simulink model "MotorJaulaArdillav2"  (R2023a)
settings: Solver=ode23s  StartTime=0.0  StopTime=1517  MaxStep=1e-3  RelTol=1e-3
PostLoadFcn:
  | load('NewCycleFTP75.mat')
  | 
  | Vel=Cycle(:,1);
  | Acc=Cycle(:,2);
InitFcn:
  | load('NewCycleFTP75.mat')
  | 
  | Vel=Cycle(:,1);
  | Acc=Cycle(:,2);
undefined symbols (not defined in the file or in its folder): sizecont
libraries: spsControlledVoltageSourceLib x3, spsAsynchronousMachineSIUnitsLib x2, dspswit3 x1, spsGroundLib x1, spsPower3phInstantaneousLib x1, spsThreePhaseVIMeasurementLib x1, spspowerguiLib x1
settings Model: SimulationMode=accelerator  Creator=ONTIBON  LastModifiedBy=Julian
settings SolverCC: ZeroCrossAlgorithm=Adaptive
settings OptimizationCC: ReuseModelBlockBuffer=off
settings DebuggingCC: IgnoredZcDiagnostic=error

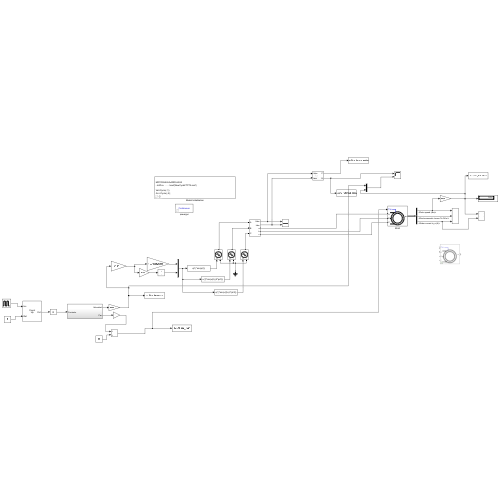
[thumbnail: Simulink's stored preview of the top-level diagram]
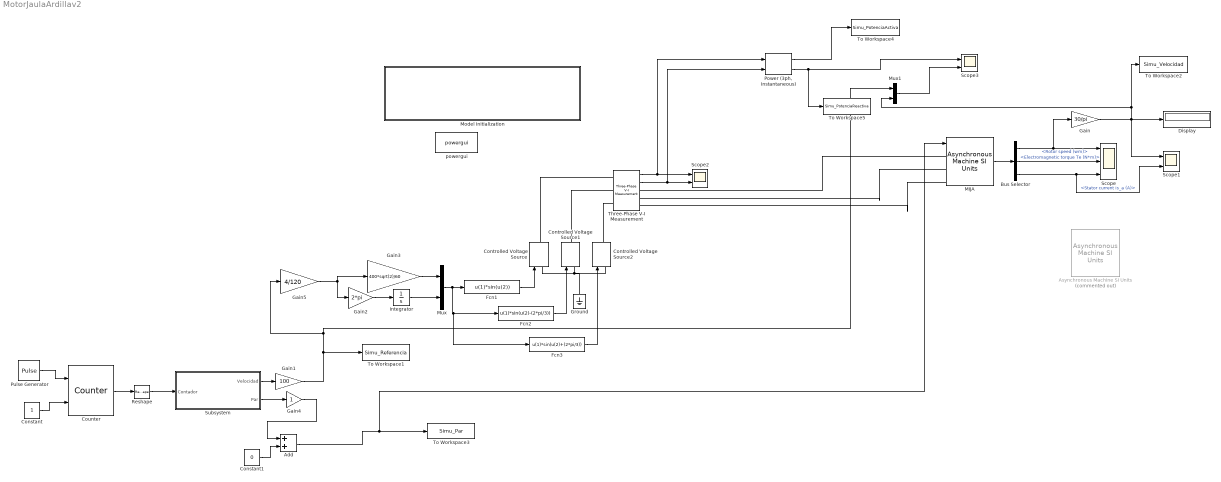
== system MotorJaulaArdillav2 ==
  Add : Sum
  Asynchronous Machine SI Units : spsAsynchronousMachineSIUnitsLib/Asynchronous Machine SI Units  Commented=on  RotorType=Squirrel-cage  PresetModel=No  MechanicalLoad=Torque Tm  ShowDetailedParameters=on  ReferenceFrame=Rotor  Units=SI  MeasurementBus=off  NominalParameters=[1.845e+04 400 50]  VoltageRatio=1  Stator=[0.5968 0.0003495]  Rotor=[0.6258 0.005473]  Cage1=[0.4155 0.002066]  Cage2=[0.4168 0.0003495]  Lm=0.0354  Mechanical=[0.05 0.005879 2]  PolePairs=2  InitialConditions=[1 0 0 0 0 0 0 0]  SimulateSaturation=off  Saturation=[14.03593122, 27.81365428, 53.79336849, 72.68890987, 97.98006896, 148.6815601, 215.7428561, 302.9841135, 428.7778367 ; 230, 322, 414, 460, 506, 552, 598, 644, 690]  LoadFlowParameters=1492000  TsPowergui=0  TsBlock=-1  IterativeModel=Trapezoidal non iterative  IterativeDiscreteModel=Trapezoidal non iterative  Pmec=1.492e+006
  Bus Selector : BusSelector  OutputSignals=Mechanical.Rotor speed (wm),Mechanical.Electromagnetic torque Te (N*m),Stator measurements.Stator current is_a (A)
  Constant : Constant
  Constant1 : Constant  Value=0
  Controlled Voltage Source : spsControlledVoltageSourceLib/Controlled Voltage Source  Initialize=on  Source_Type=AC  Amplitude=0  Phase=0  Frequency=0  Measurements=None
  Controlled Voltage Source1 : spsControlledVoltageSourceLib/Controlled Voltage Source  Initialize=on  Source_Type=AC  Amplitude=0  Phase=0  Frequency=0  Measurements=None
  Controlled Voltage Source2 : spsControlledVoltageSourceLib/Controlled Voltage Source  Initialize=on  Source_Type=AC  Amplitude=0  Phase=0  Frequency=0  Measurements=None
  Counter : dspswit3/Counter  Direction=Up  CountEvent=Rising edge  CounterSize=User defined  MaxCount=2474  InitialCount=10  Output=Count  HitValue=sizecont-1  ResetInput=on  SamplesPerFrame=1  Ts=1  CntDtype=double  HitDtype=Logical
  Display : Display
  Fcn1 : Fcn  Expr=u(1)*sin(u(2))
  Fcn2 : Fcn  Expr=u(1)*sin(u(2)-(2*pi/3))
  Fcn3 : Fcn  Expr=u(1)*sin(u(2)+(2*pi/3))
  Gain : Gain  Gain=30/pi
  Gain1 : Gain  Gain=100
  Gain2 : Gain  Gain=2*pi
  Gain3 : Gain  Gain=400*sqrt(2)/60
  Gain4 : Gain
  Gain5 : Gain  Gain=4/120
  Ground : spsGroundLib/Ground  LConnTagsString=a
  Integrator : Integrator
  MIJA : spsAsynchronousMachineSIUnitsLib/Asynchronous Machine SI Units  RotorType=Squirrel-cage  PresetModel=No  MechanicalLoad=Torque Tm  ShowDetailedParameters=on  ReferenceFrame=Rotor  Units=SI  MeasurementBus=off  NominalParameters=[250 230 50]  VoltageRatio=1  Stator=[45.50 0.20]  Rotor=[20 0.04]  Cage1=[0.4155 0.002066]  Cage2=[0.4168 0.0003495]  Lm=1.08  Mechanical=[0.03 0.0 2]  PolePairs=2  InitialConditions=[1 0 0 0 0 0 0 0]  SimulateSaturation=off  Saturation=[14.03593122, 27.81365428, 53.79336849, 72.68890987, 97.98006896, 148.6815601, 215.7428561, 302.9841135, 428.7778367 ; 230, 322, 414, 460, 506, 552, 598, 644, 690]  LoadFlowParameters=1492000  TsPowergui=0  TsBlock=-1  IterativeModel=Trapezoidal non iterative  IterativeDiscreteModel=Trapezoidal non iterative  Pmec=250
  Model Initialization : Subsystem  AncestorBlock=artemis/Tools /Misc/Model Initialization  mask(Model Functions){InitFcnX=|, prel=off, posl=on, inif=on, strf=off}
      mask InitFcnX=|
      | load('NewCycleFTP75.mat')
      |
      | Vel=Cycle(:,1);
      | Acc=Cycle(:,2);
      mask prompts: InitFcnX "Initialisation"; prel "Preload Function"; posl "PostLoad Function"; inif "InitFcn"; strf "StartFcn"
      mask init:
      | currentBlock = gcb;
      | root = bdroot(currentBlock);
      | 
      | if ~strcmp(get_param(root,'BlockDiagramType'),'library')
      |     if prel==1
      |         set_param(root, 'PreLoadFcn', InitFcnX);
      |     else
      |         set_param(root, 'PreLoadFcn', '');
      |     end
      |     if inif==1
      |         set_param(root, 'InitFcn', InitFcnX);
      |     else
      |         set_param(root, 'InitFcn', '');
      |     end
      |     if strf==1
      |         set_param(root, 'StartFcn', InitFcnX);
      |     else
      |         set_param(root, 'StartFcn', '');
      |     end
      |     if posl==1
      |         set_param(root, 'PostLoadFcn', InitFcnX);
      |     else
      |         set_param(root, 'PostLoadFcn', '');
      |     end
      | end
      | 
      | pos = get_param(currentBlock, 'Position');
      | width = pos(3) - pos(1); height = pos(4) - pos(2);
      | txt = [ upper(root) '\n' '- InitFcn. . . . . '  get_param(root, 'InitFcn') ];
      settings: LibrarySourceBlock=artemis/Tools /Misc/Model Initialization  CopyFcn=set_param(gcb,'LinkStatus','inactive')
      mask Display: text(5, height*0.5, txt, 'horizontalAlignment', 'left', 'verticalAlignment', 'middle') ;
  Mux : Mux  Inputs=2
  Mux1 : Mux  Inputs=2
  "Power (3ph, Instantaneous)" : spsPower3phInstantaneousLib/Power (3ph, Instantaneous)
  Pulse Generator : DiscretePulseGenerator  PulseType=Time based  Period=1  PulseWidth=5
  Reshape : Reshape  OutputDimensionality=Customize  OutputDimensions=[1]
  Scope : Scope  NumInputPorts=3
  Scope1 : Scope  NumInputPorts=2
  Scope2 : Scope  NumInputPorts=2
  Scope3 : Scope  NumInputPorts=2
  Subsystem : Subsystem
  Three-Phase V-I Measurement : spsThreePhaseVIMeasurementLib/Three-Phase V-I Measurement  VoltageMeasurement=phase-to-ground  SetLabelV=off  LabelV=Vabc  Vpu=off  VpuLL=off  CurrentMeasurement=yes  SetLabelI=off  LabelI=Iabc  Ipu=off  Pbase=100e6  Vbase=500e3  OutputType=Complex  PhasorSimulation=off  PSBequivalent=0
  To Workspace1 : ToWorkspace  VariableName=Simu_Referencia  SampleTime=1/2000
      settings: Save2DSignal=2-D array (concatenate along first dimension)
  To Workspace2 : ToWorkspace  VariableName=Simu_Velocidad  SampleTime=1/2000
      settings: Save2DSignal=2-D array (concatenate along first dimension)
  To Workspace3 : ToWorkspace  VariableName=Simu_Par  SampleTime=1/2000
      settings: Save2DSignal=2-D array (concatenate along first dimension)
  To Workspace4 : ToWorkspace  VariableName=Simu_PotenciaActiva  SampleTime=1/2000
      settings: Save2DSignal=2-D array (concatenate along first dimension)
  To Workspace5 : ToWorkspace  VariableName=Simu_PotenciaReactiva  SampleTime=1/2000
      settings: Save2DSignal=2-D array (concatenate along first dimension)
  powergui : spspowerguiLib/powergui  Priority=1  SimulationMode=Continuous  SampleTime=50e-6  frequency=60  Iterations=50  frequencyindice=50  Pbase=100e6  ErrMax=1e-4  UnitsV=kV  UnitsW=MW  buscounter=0  FunctionMessages=off  echomessages=off  EnableUseOfTLC=off  CurrentSourceSwitches=off  DisableSnubberDevices=off  DisableRonSwitches=off  DisableVfSwitches=off  DisplayEquations=off  AutomaticDiscreteSolvers=off  SolverType=Tustin/Backward Euler (TBE)  Interpol=off  ExternalGateDelay=off  methode=off  Ts=100  x0status=blocks  SPID=on  SwTol=0  HookPort=off  NonlinearTolerance=1e-4  nMaxIteration=100  ContinueOnMaxIteration=off  RestoreLinks=warning  ResistiveCurrentMeasurement=off  Frange=[0:2:500]  Ylog=off  Xlog=on  ShowGrid=off  save=off  variable=ZData  structure=0  ZoomFFT=off  StartTime=0.0  cycles=1  DisplayStyle=1  fundamental=60  FreqAxis=off  MaxFrequency=1000  frequencyindicesteady=1  RmsSteady=1  display=off
  wires:
  MIJA/1 -> Bus Selector/1
  Gain/1 -> To Workspace2/1, Mux1/2, Scope1/1, Display/1
  Bus Selector/1 -> Gain/1, Scope/1  "<Rotor speed (wm)>"
  Bus Selector/2 -> Scope/2  "<Electromagnetic torque Te (N*m)>"
  Bus Selector/3 -> Scope1/2, Scope/3  "<Stator current is_a (A)>"
  Fcn1/1 -> Controlled Voltage Source/1
  Fcn2/1 -> Controlled Voltage Source1/1
  Fcn3/1 -> Controlled Voltage Source2/1
  Mux/1 -> Fcn3/1, Fcn2/1, Fcn1/1
  Integrator/1 -> Mux/2
  Gain2/1 -> Integrator/1
  Gain3/1 -> Mux/1
  Gain1/1 -> Mux1/1, Gain5/1, To Workspace1/1
  Three-Phase V-I Measurement/2 -> "Power (3ph, Instantaneous)"/2, Scope2/2
  Three-Phase V-I Measurement/1 -> "Power (3ph, Instantaneous)"/1, Scope2/1
  "Power (3ph, Instantaneous)"/2 -> To Workspace5/1, Scope3/1
  Subsystem/2(Par) -> Gain4/1
  Subsystem/1(Velocidad) -> Gain1/1
  Pulse Generator/1 -> Counter/1
  Counter/1 -> Reshape/1
  Reshape/1 -> Subsystem/1(Contador)
  Constant/1 -> Counter/2
  Gain4/1 -> Add/1
  Mux1/1 -> Scope3/2
  Gain5/1 -> Gain3/1, Gain2/1
  "Power (3ph, Instantaneous)"/1 -> To Workspace4/1
  Constant1/1 -> Add/2
  Add/1 -> MIJA/1, To Workspace3/1
  connections:
  Controlled Voltage Source/LConn1 -- Ground/LConn1 -- Controlled Voltage Source2/LConn1 -- Controlled Voltage Source1/LConn1
  Three-Phase V-I Measurement/LConn3 -- Controlled Voltage Source2/RConn1
  Three-Phase V-I Measurement/LConn2 -- Controlled Voltage Source1/RConn1
  Three-Phase V-I Measurement/LConn1 -- Controlled Voltage Source/RConn1
  MIJA/LConn1 -- Three-Phase V-I Measurement/RConn1
  MIJA/LConn2 -- Three-Phase V-I Measurement/RConn2
  MIJA/LConn3 -- Three-Phase V-I Measurement/RConn3

== system MotorJaulaArdillav2/Model Initialization ==

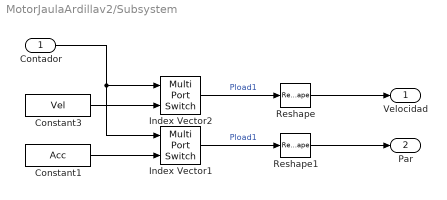
== system MotorJaulaArdillav2/Subsystem ==
  Contador : Inport
  Constant1 : Constant  Value=Acc
  Constant3 : Constant  Value=Vel
  Index Vector1 : MultiPortSwitch  DataPortOrder=Zero-based contiguous  Inputs=1  zeroidx=on  SaturateOnIntegerOverflow=off  InputSameDT=off
  Index Vector2 : MultiPortSwitch  DataPortOrder=Zero-based contiguous  Inputs=1  zeroidx=on  SaturateOnIntegerOverflow=off  InputSameDT=off
  Reshape : Reshape  OutputDimensionality=Customize  OutputDimensions=[1]
  Reshape1 : Reshape  OutputDimensionality=Customize  OutputDimensions=[1]
  Velocidad : Outport
  Par : Outport  Port=2
  wires:
  Constant3/1 -> Index Vector2/2
  Index Vector1/1 -> Reshape1/1  "Pload1"
  Index Vector2/1 -> Reshape/1  "Pload1"
  Reshape1/1 -> Par/1
  Reshape/1 -> Velocidad/1
  Constant1/1 -> Index Vector1/2
  Contador/1 -> Index Vector2/1, Index Vector1/1
